simulink model "RightForceSensorAgent"  (Simulink 6.2)
settings: Solver=ode45  SolverMode=SingleTasking  StartTime=0.0  StopTime=10.0  RelTol=1e-3  AbsTol=1e-6
settings Model: Creator=The MathWorks Inc.  LastModifiedBy=suarezjl  ExtModeTrigMode=oneshot  ExtModeArmWhenConnect=off  ExtModeAutoUpdateStatusClock=off
settings DataIOCC: LimitDataPoints=off  SignalLoggingName=logsOut
settings OptimizationCC: BooleanDataType=off  InlineInvariantSignals=on
settings DebuggingCC: CheckExecutionContextPreStartOutputMsg=on  CheckExecutionContextRuntimeOutputMsg=on  IntegerOverflowMsg=none
settings HardwareCC: TargetUnknown=on
settings ModelReferenceCC: UpdateModelReferenceTargets=IfOutOfDate

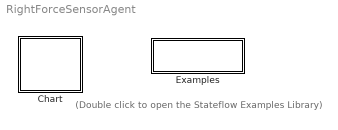
== system RightForceSensorAgent ==
  note: (Double click to open the
      | Stateflow Examples Library)
  Chart : Stateflow chart
  Examples : Subsystem
      settings: OpenFcn=sf('Private','sf_examples')
      mask Display: disp('Examples')

== system RightForceSensorAgent/Examples ==

== stateflow chart Chart ==
  state Initialize
    \\Octavia\ISACControlBasisModule\RightModule\ForceSensor\ATISensor.Initialize()
  state ReadFTData
    \\Octavia\ISACControlBasisModule\RightModule\ForceSensor\ATISensor.SampleFTData()
  state Stop
  (default) -> Initialize : Start
  Initialize -> ReadFTData : Always
  ReadFTData -> ReadFTData [order 1] : Default
  ReadFTData -> Stop [order 2] : Signal="End"
